simulink model "portret"  (R2024b)
settings: Solver=VariableStepAuto  StartTime=0.0  StopTime=1150  MaxStep=0.01  RelTol=1e-3
values from neighbouring files (symbols this model uses):
  czas_skok = 0    [portret_fazowy.m]
  u_0 = 1    [portret_fazowy.m]
  u_1 = 10    [portret_fazowy.m]
  w_n = 3    [portret_fazowy.m]
  x_0 = stany_pocz_x(k)    [portret_fazowy.m]
  x_dot_0 = stany_pocz_x_dot(k)    [portret_fazowy.m]
  xi = roz_xi(i)    [portret_fazowy.m]
settings Model: Creator=userbrigh  LastModifiedBy=userbrigh

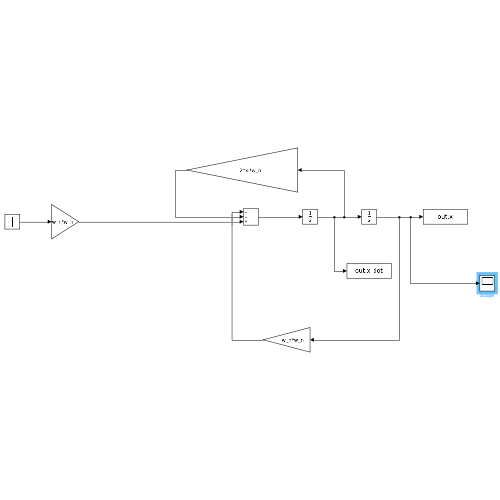
[thumbnail: Simulink's stored preview of the top-level diagram]
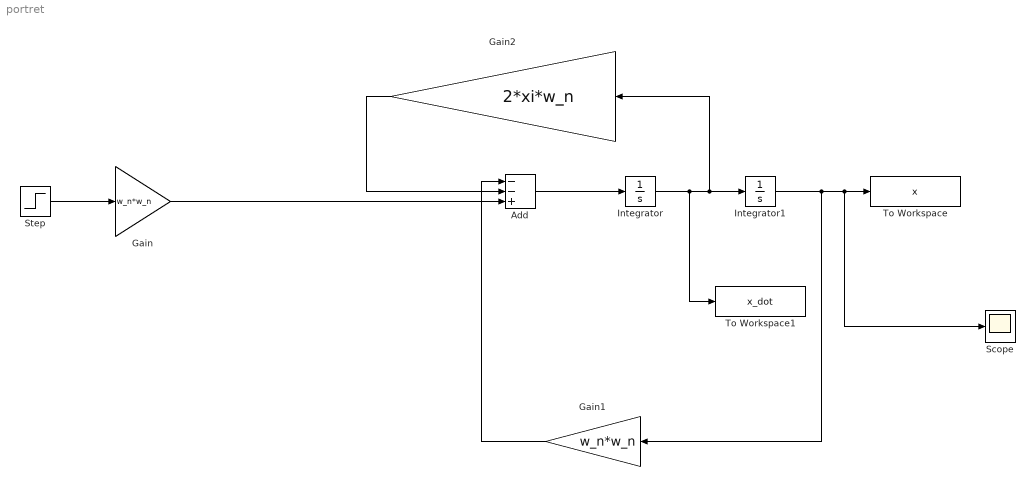
== system portret ==
  Add : Sum  Inputs=--+
  Gain : Gain  Gain=w_n*w_n
  Gain1 : Gain  Gain=w_n*w_n
  Gain2 : Gain  Gain=2*xi*w_n
  Integrator : Integrator  InitialCondition=x_dot_0
  Integrator1 : Integrator  InitialCondition=x_0
  Scope : Scope
  Step : Step  Time=czas_skok  Before=u_0  After=u_0+u_1  SampleTime=0
  To Workspace : ToWorkspace  VariableName=x  SampleTime=-1
  To Workspace1 : ToWorkspace  VariableName=x_dot  SampleTime=-1
  wires:
  Integrator/1 -> To Workspace1/1, Gain2/1, Integrator1/1
  Integrator1/1 -> Gain1/1, Scope/1, To Workspace/1
  Step/1 -> Gain/1
  Gain/1 -> Add/3
  Add/1 -> Integrator/1
  Gain1/1 -> Add/1
  Gain2/1 -> Add/2
